simulink subsystem "Lat_Dir_Aero_Forces_Moments"  (R2025b)
settings: Solver=VariableStepAuto  StartTime=0.0  StopTime=10.0  RelTol=1e-3
undefined symbols (not defined in the file): CL_delAil, CL_delRud, CL_p, CL_r, CN_beta, CN_delAil, CN_delRud, CN_p, CN_r, CY_beta, CY_beta_dot, CY_delAil, CY_delRud, CY_p, CY_r, p0, r0, Span, Sref, u0, U1
libraries: simulink_extras x2
settings Model: Creator=cdriggs  LastModifiedBy=Ky Bui

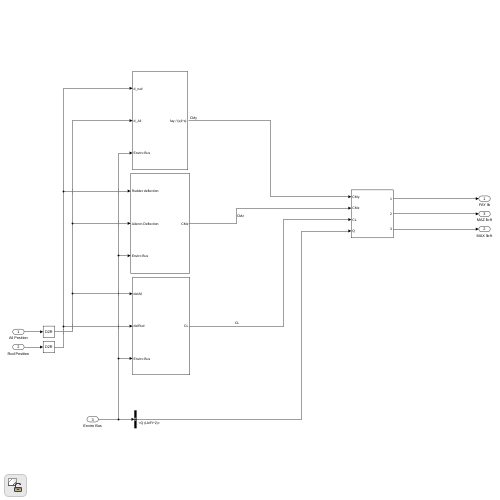
[thumbnail: Simulink's stored preview of the top-level diagram]
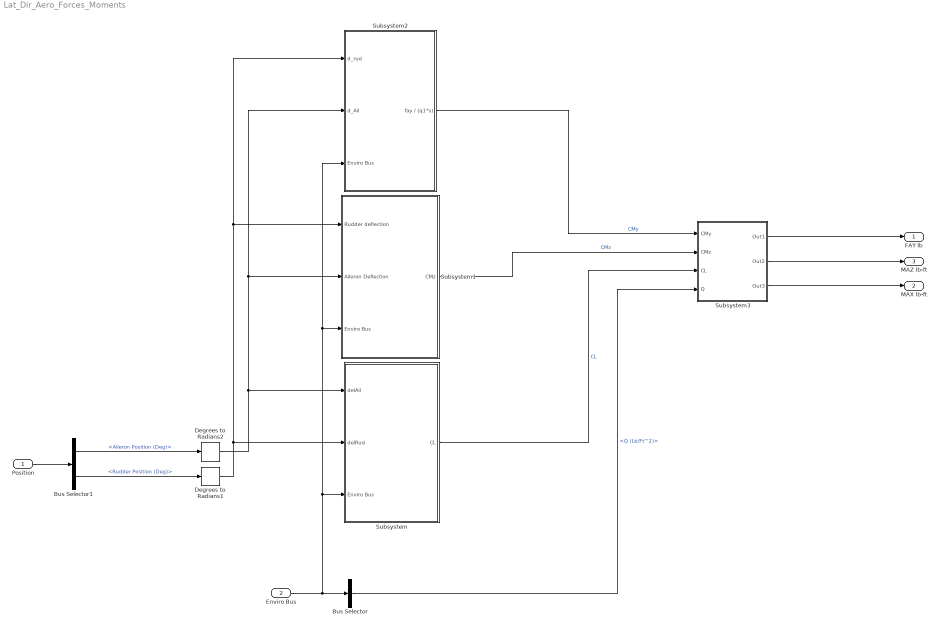
== system Lat_Dir_Aero_Forces_Moments ==
  Position : Inport
  Enviro Bus : Inport  Port=2
  Bus Selector : BusSelector  OutputSignals=Q (Lb/Ft^2)
  Bus Selector1 : BusSelector  OutputSignals=Aileron Position (Deg),Rudder Position (Deg)
  Degrees to Radians1 : simulink_extras/Transformations/Degrees to Radians
  Degrees to Radians2 : simulink_extras/Transformations/Degrees to Radians
  Subsystem : Subsystem
  Subsystem1 : Subsystem
  Subsystem2 : Subsystem
  Subsystem3 : Subsystem
  FAY lb : Outport
  MAX lb-ft : Outport  Port=2
  MAZ lb-ft : Outport  Port=3
  wires:
  Enviro Bus/1 -> Bus Selector/1, Subsystem/3(Enviro Bus), Subsystem1/3(Enviro Bus), Subsystem2/3(Enviro Bus)
  Subsystem2/1(fay / (q1*s)) -> Subsystem3/1(CMy)  "CMy"
  Subsystem1/1(CMz) -> Subsystem3/2(CMz)  "CMz"
  Bus Selector/1 -> Subsystem3/4("Q ")  "<Q (Lb/Ft^2)>"
  Subsystem/1(CL) -> Subsystem3/3(CL)  "CL"
  Subsystem3/1(Out1) -> FAY lb/1
  Subsystem3/2(Out2) -> MAZ lb-ft/1
  Subsystem3/3(Out3) -> MAX lb-ft/1
  Degrees to Radians2/1 -> Subsystem/1(delAil), Subsystem1/2(Aileron Deflection), Subsystem2/2(d_Ail)
  Degrees to Radians1/1 -> Subsystem/2(delRud), Subsystem1/1(Rudder deflection), Subsystem2/1(d_rud)
  Position/1 -> Bus Selector1/1
  Bus Selector1/2 -> Degrees to Radians1/1  "<Rudder Position (Deg)>"
  Bus Selector1/1 -> Degrees to Radians2/1  "<Aileron Position (Deg)>"

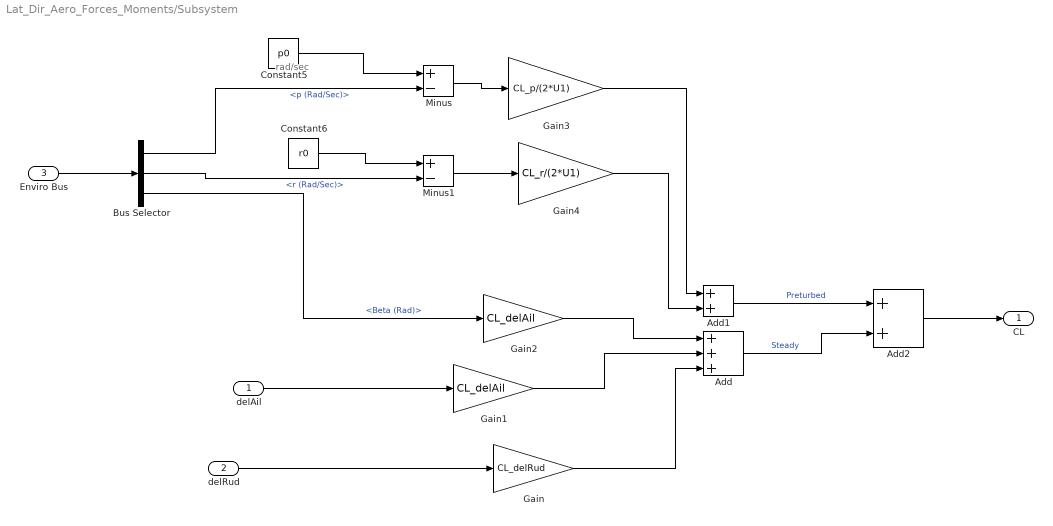
== system Lat_Dir_Aero_Forces_Moments/Subsystem ==
  note: rad/sec
  delAil : Inport
  delRud : Inport  Port=2
  Enviro Bus : Inport  Port=3
  Add : Sum  Inputs=+++
  Add1 : Sum
  Add2 : Sum
  Bus Selector : BusSelector  OutputSignals=Rotat.Body.Rates (Rad/Sec).p (Rad/Sec),Rotat.Body.Rates (Rad/Sec).r (Rad/Sec),Aero angles.Beta (Rad)
  Constant5 : Constant  Value=p0
  Constant6 : Constant  Value=r0
  Gain : Gain  Gain=CL_delRud
  Gain1 : Gain  Gain=CL_delAil
  Gain2 : Gain  Gain=CL_delAil
  Gain3 : Gain  Gain=CL_p/(2*U1)
  Gain4 : Gain  Gain=CL_r/(2*U1)
  Minus : Sum  Inputs=+-
  Minus1 : Sum  Inputs=+-
  CL : Outport
  wires:
  Enviro Bus/1 -> Bus Selector/1
  Gain4/1 -> Add1/2
  Minus1/1 -> Gain4/1
  Minus/1 -> Gain3/1
  Bus Selector/1 -> Minus/2  "<p (Rad/Sec)>"
  Gain2/1 -> Add/1
  Bus Selector/3 -> Gain2/1  "<Beta (Rad)>"
  Gain1/1 -> Add/2
  delAil/1 -> Gain1/1
  Gain/1 -> Add/3
  Constant6/1 -> Minus1/1
  Add2/1 -> CL/1
  Bus Selector/2 -> Minus1/2  "<r (Rad/Sec)>"
  delRud/1 -> Gain/1
  Constant5/1 -> Minus/1
  Add/1 -> Add2/2  "Steady"
  Gain3/1 -> Add1/1
  Add1/1 -> Add2/1  "Preturbed"

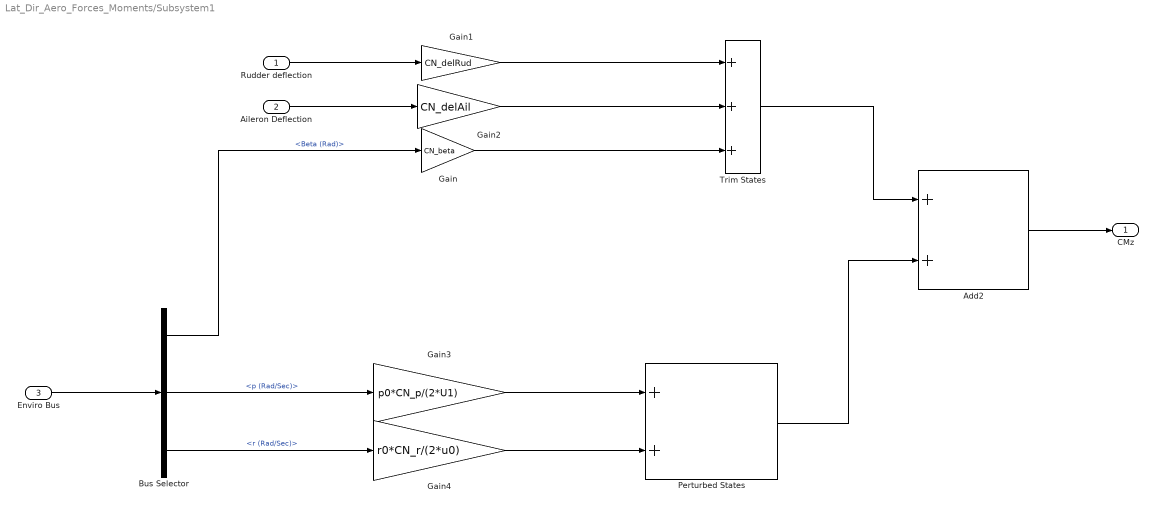
== system Lat_Dir_Aero_Forces_Moments/Subsystem1 ==
  Rudder deflection : Inport
  Aileron Deflection : Inport  Port=2
  Enviro Bus : Inport  Port=3
  Add2 : Sum
  Bus Selector : BusSelector  OutputSignals=Aero angles.Beta (Rad),Rotat.Body.Rates (Rad/Sec).p (Rad/Sec),Rotat.Body.Rates (Rad/Sec).r (Rad/Sec)
  Gain : Gain  Gain=CN_beta
  Gain1 : Gain  Gain=CN_delRud
  Gain2 : Gain  Gain=CN_delAil
  Gain3 : Gain  Gain=p0*CN_p/(2*U1)
  Gain4 : Gain  Gain=r0*CN_r/(2*u0)
  Perturbed States : Sum
  Trim States : Sum  Inputs=+++
  CMz : Outport
  wires:
  Gain/1 -> Trim States/3
  Bus Selector/1 -> Gain/1  "<Beta (Rad)>"
  Enviro Bus/1 -> Bus Selector/1
  Bus Selector/3 -> Gain4/1  "<r (Rad/Sec)>"
  Bus Selector/2 -> Gain3/1  "<p (Rad/Sec)>"
  Aileron Deflection/1 -> Gain2/1
  Gain1/1 -> Trim States/1
  Rudder deflection/1 -> Gain1/1
  Gain4/1 -> Perturbed States/2
  Trim States/1 -> Add2/1
  Gain3/1 -> Perturbed States/1
  Gain2/1 -> Trim States/2
  Add2/1 -> CMz/1
  Perturbed States/1 -> Add2/2

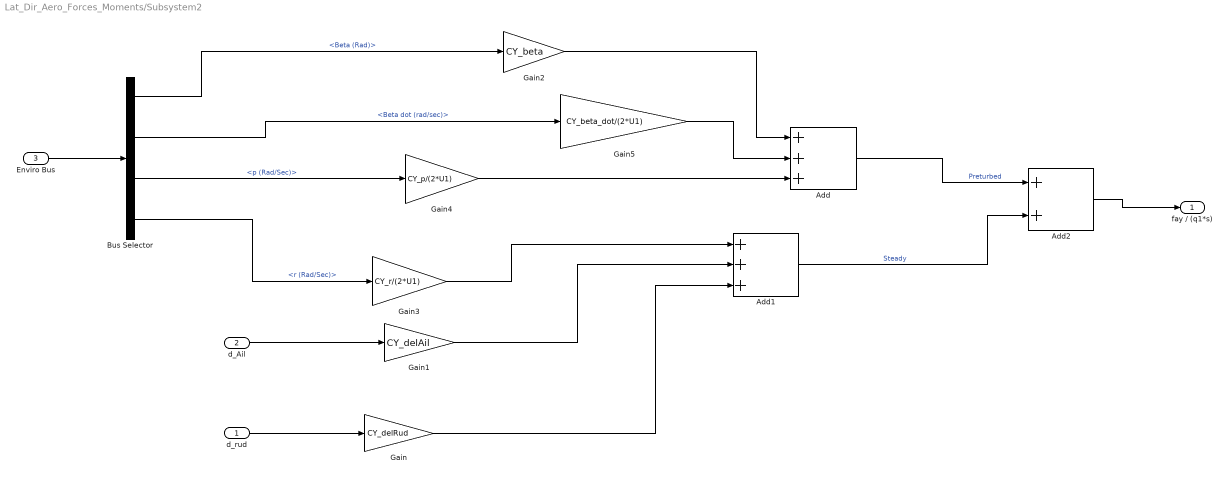
== system Lat_Dir_Aero_Forces_Moments/Subsystem2 ==
  d_rud : Inport
  d_Ail : Inport  Port=2
  Enviro Bus : Inport  Port=3
  Add : Sum  Inputs=+++
  Add1 : Sum  Inputs=+++
  Add2 : Sum
  Bus Selector : BusSelector  OutputSignals=Aero angles.Beta (Rad),Aero angles.Beta dot (rad/sec),Rotat.Body.Rates (Rad/Sec).p (Rad/Sec),Rotat.Body.Rates (Rad/Sec).r (Rad/Sec)
  Gain : Gain  Gain=CY_delRud
  Gain1 : Gain  Gain=CY_delAil
  Gain2 : Gain  Gain=CY_beta
  Gain3 : Gain  Gain=CY_r/(2*U1)
  Gain4 : Gain  Gain=CY_p/(2*U1)
  Gain5 : Gain  Gain=CY_beta_dot/(2*U1)
  fay / (q1*s) : Outport
  wires:
  Enviro Bus/1 -> Bus Selector/1
  Gain5/1 -> Add/2
  Gain4/1 -> Add/3
  Bus Selector/3 -> Gain4/1  "<p (Rad/Sec)>"
  Bus Selector/4 -> Gain3/1  "<r (Rad/Sec)>"
  Gain2/1 -> Add/1
  Gain1/1 -> Add1/2
  d_Ail/1 -> Gain1/1
  Gain/1 -> Add1/3
  d_rud/1 -> Gain/1
  Bus Selector/1 -> Gain2/1  "<Beta (Rad)>"
  Gain3/1 -> Add1/1
  Add1/1 -> Add2/2  "Steady"
  Add2/1 -> fay / (q1*s)/1
  Bus Selector/2 -> Gain5/1  "<Beta dot (rad/sec)>"
  Add/1 -> Add2/1  "Preturbed"

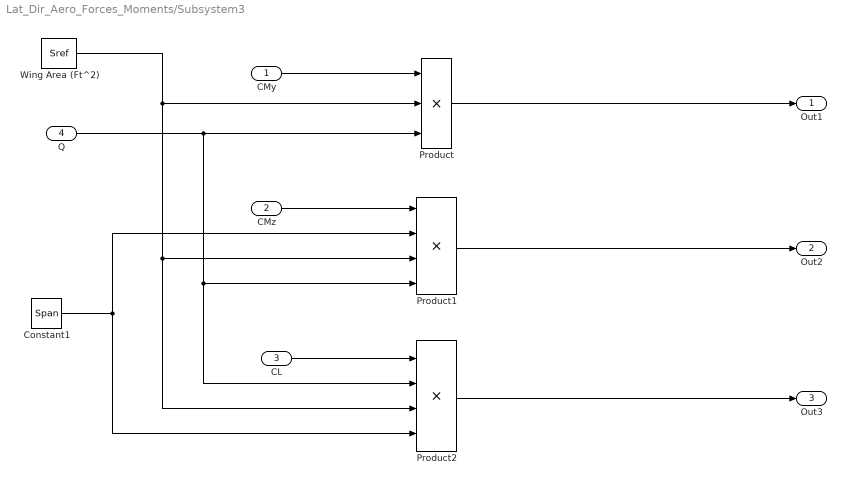
== system Lat_Dir_Aero_Forces_Moments/Subsystem3 ==
  CMy : Inport
  CMz : Inport  Port=2
  CL : Inport  Port=3
  "Q " : Inport  Port=4
  Constant1 : Constant  Value=Span
  Product : Product  Inputs=3
  Product1 : Product  Inputs=****
  Product2 : Product  Inputs=4
  Wing Area (Ft^2) : Constant  Value=Sref
  Out1 : Outport
  Out2 : Outport  Port=2
  Out3 : Outport  Port=3
  wires:
  Constant1/1 -> Product1/2, Product2/4
  "Q "/1 -> Product/3, Product1/4, Product2/2
  CMz/1 -> Product1/1
  Product2/1 -> Out3/1
  Wing Area (Ft^2)/1 -> Product/2, Product1/3, Product2/3
  Product/1 -> Out1/1
  Product1/1 -> Out2/1
  CL/1 -> Product2/1
  CMy/1 -> Product/1
